simulink model "flyback_dt_antiwindup"  (R2021b)
settings: Solver=FixedStepAuto  StartTime=0.0  StopTime=10  RelTol=1e-3
undefined symbols (not defined in the file): DiscIntNeverNeededParam
Description:
  | Symmetric FIR Filter
  | This example shows how to use HDL Coder(TM) to check, generate,
  | and verify HDL for a fixed-point symmetric FIR filter.
settings Model: DataTypeOverride=Off  Creator=The MathWorks, Inc.  LastModifiedBy=Marco Milanesi
settings SolverCC: AlgebraicLoopSolver=TrustRegion  AutoInsertRateTranBlk=on
settings DataIOCC: LimitDataPoints=on  SaveFormat=Array  SaveOutput=off  SignalLogging=off  SaveTime=off  ReturnWorkspaceOutputs=off  SignalLoggingName=logsOut
settings OptimizationCC: BlockReduction=off  BooleanDataType=off  ConditionallyExecuteInputs=off  DefaultParameterBehavior=Inlined  InheritOutputTypeSmallerThanSingle=on  InlineInvariantSignals=on  ExpressionDepthLimit=2147483647  InitFltsAndDblsToZero=on  LifeSpan=inf  BufferReusableBoundary=off
settings DebuggingCC: AlgebraicLoopMsg=error  SaveWithParameterizedLinksMsg=none  UnderspecifiedInitializationDetection=Classic  MergeDetectMultiDrivingBlocksExec=none  CheckExecutionContextPreStartOutputMsg=on  SignalResolutionControl=TryResolveAllWithWarning  MultiTaskDSMMsg=warning  MultiTaskCondExecSysMsg=none  SingleTaskRateTransMsg=error  IntegerOverflowMsg=none  ParameterPrecisionLossMsg=none  FcnCallInpInsideContextMsg=warning  BusObjectLabelMismatch=none  StateNameClashWarn=warning  SFUnexpectedBacktrackingDiag=warning  SFNoUnconditionalDefaultTransitionDiag=warning  SFExecutionAtInitializationDiag=none  SFMachineParentedDataDiag=warning  IntegerSaturationMsg=none  ArithmeticOperatorsInVariantConditions=warning
settings HardwareCC: ProdBitPerPointer=32  ProdBitPerSizeT=32  ProdBitPerPtrDiffT=32  ProdLargestAtomicFloat=None  ProdIntDivRoundTo=Undefined  ProdEndianess=Unspecified  ProdWordSize=32  ProdHWDeviceType=ASIC/FPGA  TargetUnknown=on  ProdEqTarget=off
settings ModelReferenceCC: PropagateSignalLabelsOutOfModel=off
settings SFSimCC: SimUseLocalCustomCode=off  CustomCodeUndefinedFunction=UseInterfaceOnly
settings RTWCC: RTWUseLocalCustomCode=off
settings CodeAppCC: StateflowObjectComments=on
settings GRTTargetCC: TargetFcnLib=ansi_tfl_tmw.mat  TargetLangStandard=C89/C90 (ANSI)  CombineOutputUpdateFcns=off  GRTInterface=on
settings ConfigComp: CovMetricSettings=dw  CovSaveCumulativeToWorkspaceVar=on  CovSaveSingleToWorkspaceVar=on  CovExternalEMLEnable=off

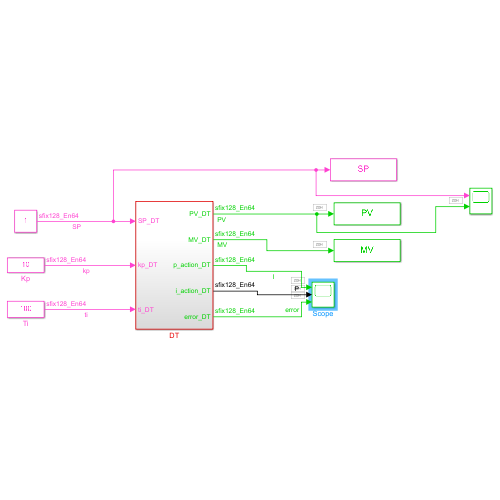
[thumbnail: Simulink's stored preview of the top-level diagram]
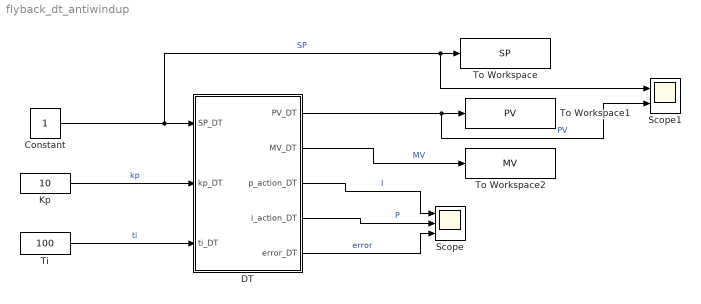
== system flyback_dt_antiwindup ==
  Constant : Constant  OutDataTypeStr=fixdt(1,128,64)
  DT : Subsystem
  Kp : Constant  Value=10  OutDataTypeStr=fixdt(1,128,64)
  Scope : Scope  NumInputPorts=3
  Scope1 : Scope  NumInputPorts=2
  Ti : Constant  Value=100  OutDataTypeStr=fixdt(1,128,64)
  To Workspace : ToWorkspace  VariableName=SP  SaveFormat=Structure With Time  SampleTime=-1
  To Workspace1 : ToWorkspace  VariableName=PV  SaveFormat=Structure With Time  SampleTime=-1
  To Workspace2 : ToWorkspace  VariableName=MV  SaveFormat=Structure With Time  SampleTime=-1
  wires:
  Kp/1 -> DT/2(kp_DT)  "kp"
  Ti/1 -> DT/3(ti_DT)  "ti"
  Constant/1 -> Scope1/1, To Workspace/1, DT/1(SP_DT)  "SP"
  DT/3(p_action_DT) -> Scope/1  "I"
  DT/5(error_DT) -> Scope/3  "error"
  DT/1(PV_DT) -> Scope1/2, To Workspace1/1  "PV"
  DT/2(MV_DT) -> To Workspace2/1  "MV"
  DT/4(i_action_DT) -> Scope/2  "P"

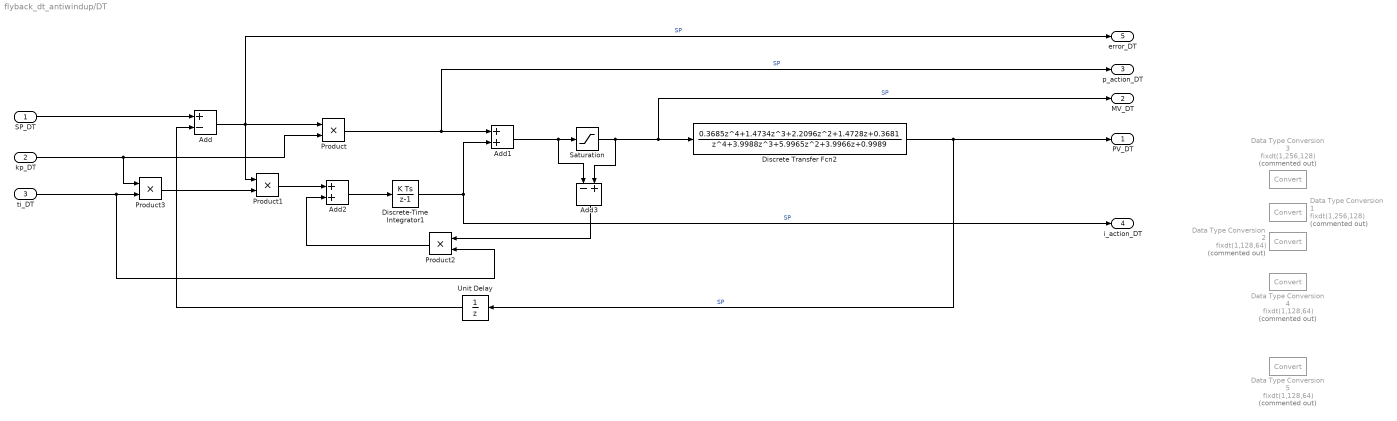
== system flyback_dt_antiwindup/DT ==
  SP_DT : Inport
  kp_DT : Inport  Port=2
  ti_DT : Inport  Port=3
  Add : Sum  Inputs=+-  AccumDataTypeStr=fixdt(1,128,64)  OutDataTypeStr=fixdt(1,128,64)
  Add1 : Sum  AccumDataTypeStr=fixdt(1,128,64)  OutDataTypeStr=fixdt(1,128,64)
  Add2 : Sum  AccumDataTypeStr=fixdt(1,128,64)  OutDataTypeStr=fixdt(1,128,64)
  Add3 : Sum  Inputs=-+  AccumDataTypeStr=fixdt(1,128,64)  OutDataTypeStr=fixdt(1,128,64)
  Data Type Conversion1 : DataTypeConversion  Commented=on  OutDataTypeStr=fixdt(1,256,128)
  Data Type Conversion2 : DataTypeConversion  Commented=on  OutDataTypeStr=fixdt(1,128,64)
  Data Type Conversion3 : DataTypeConversion  Commented=on  OutDataTypeStr=fixdt(1,256,128)
  Data Type Conversion4 : DataTypeConversion  Commented=on  OutDataTypeStr=fixdt(1,128,64)
  Data Type Conversion5 : DataTypeConversion  Commented=on  OutDataTypeStr=fixdt(1,128,64)
  Discrete Transfer Fcn2 : DiscreteTransferFcn  Numerator=[0.3685 1.4734 2.2096 1.4728 0.3681]  Denominator=[1 3.9988 5.9965 3.9966 0.9989]  SampleTime=0.00001  NumCoefDataTypeStr=fixdt(1,128,64)  DenCoefDataTypeStr=fixdt(1,128,64)  NumProductDataTypeStr=fixdt(1,128,64)  DenProductDataTypeStr=fixdt(1,128,64)  NumAccumDataTypeStr=fixdt(1,128,64)  DenAccumDataTypeStr=fixdt(1,128,64)  OutDataTypeStr=fixdt(1,128,64)
  Discrete-Time Integrator1 : DiscreteIntegrator  SampleTime=0.00001  OutDataTypeStr=fixdt(1,128,64)  ICPrevOutput=DiscIntNeverNeededParam  ICPrevScaledInput=DiscIntNeverNeededParam
  Product{,1..3} (4 alike) : Product  OutDataTypeStr=fixdt(1,128,64)
  Saturation : Saturate  UpperLimit=255  LowerLimit=-255  OutDataTypeStr=fixdt(1,128,64)
  Unit Delay : UnitDelay  SampleTime=0.00001  HasFrameUpgradeWarning=on
  PV_DT : Outport  OutDataTypeStr=fixdt(1,128,64)  SampleTime=0.001  VectorParamsAs1DForOutWhenUnconnected=off
  MV_DT : Outport  Port=2  OutDataTypeStr=fixdt(1,128,64)  SampleTime=0.001  VectorParamsAs1DForOutWhenUnconnected=off
  p_action_DT : Outport  Port=3  OutDataTypeStr=fixdt(1,128,64)  SampleTime=0.001  VectorParamsAs1DForOutWhenUnconnected=off
  i_action_DT : Outport  Port=4  OutDataTypeStr=fixdt(1,128,64)  SampleTime=0.001  VectorParamsAs1DForOutWhenUnconnected=off
  error_DT : Outport  Port=5  OutDataTypeStr=fixdt(1,128,64)  SampleTime=0.001  VectorParamsAs1DForOutWhenUnconnected=off
  wires:
  SP_DT/1 -> Add/1
  kp_DT/1 -> Product/2, Product3/1
  Unit Delay/1 -> Add/2
  Add1/1 -> Add3/1, Saturation/1
  Product1/1 -> Add2/1
  Add2/1 -> Discrete-Time Integrator1/1
  Add3/1 -> Product2/1
  Product2/1 -> Add2/2
  ti_DT/1 -> Product3/2, Product2/2
  Product3/1 -> Product1/2
  Add/1 -> error_DT/1, Product/1, Product1/1  "SP"
  Product/1 -> p_action_DT/1, Add1/1  "SP"
  Discrete Transfer Fcn2/1 -> PV_DT/1, Unit Delay/1  "SP"
  Saturation/1 -> MV_DT/1, Discrete Transfer Fcn2/1, Add3/2  "SP"
  Discrete-Time Integrator1/1 -> i_action_DT/1, Add1/2  "SP"
